simulink model "ATABEY_sistem_modeli"  (R2025b)
settings: Solver=VariableStepAuto  StartTime=0.0  StopTime=simTime  RelTol=1e-3
undefined symbols (not defined in the file or in its folder): uServoMax, x0
libraries: aerolibfltsims x1, aerolibanimutils x1
settings Model: Creator=erayacikgz  LastModifiedBy=erayacikgz

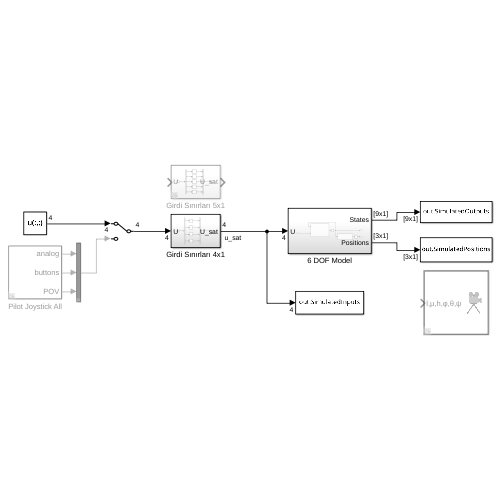
[thumbnail: Simulink's stored preview of the top-level diagram]
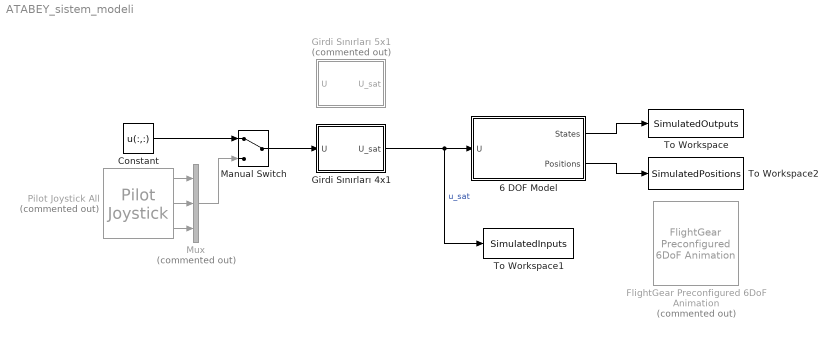
== system ATABEY_sistem_modeli ==
  6 DOF Model : Subsystem
  Constant : Constant  Value=u(:,:)
  FlightGear Preconfigured 6DoF Animation : aerolibfltsims/FlightGear Preconfigured 6DoF Animation  Commented=on  xFlightGearVersion=v2019.1  DestinationIpAddress=127.0.0.1  DestinationPort=5502  SampleTime=1/30  packetVersion=24
  Girdi Sınırları 4x1 : Subsystem
  Girdi Sınırları 5x1 : Subsystem  Commented=on
  Manual Switch : ManualSwitch
  Mux : Mux  Commented=on  Inputs=3
  Pilot Joystick All : aerolibanimutils/Pilot Joystick  Commented=on  JoystickID=Joystick1  OutputConfiguration=AllOutputs  SampleTime=1/30
      settings: LibrarySourceBlock=aerolibanimutils/Pilot Joystick All
  To Workspace : ToWorkspace  VariableName=SimulatedOutputs  SaveFormat=Timeseries  SampleTime=-1
  To Workspace1 : ToWorkspace  VariableName=SimulatedInputs  SaveFormat=Timeseries  SampleTime=-1
  To Workspace2 : ToWorkspace  VariableName=SimulatedPositions  SaveFormat=Timeseries  SampleTime=-1
  wires:
  6 DOF Model/1(States) -> To Workspace/1
  Constant/1 -> Manual Switch/1
  Pilot Joystick All/1 -> Mux/1
  Pilot Joystick All/2 -> Mux/2
  Pilot Joystick All/3 -> Mux/3
  Mux/1 -> Manual Switch/2
  6 DOF Model/2(Positions) -> To Workspace2/1
  Manual Switch/1 -> Girdi Sınırları 4x1/1(U)
  Girdi Sınırları 4x1/1(U_sat) -> To Workspace1/1, 6 DOF Model/1(U)  "u_sat"

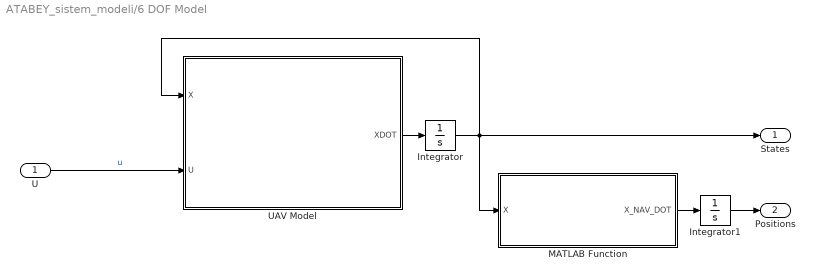
== system ATABEY_sistem_modeli/6 DOF Model ==
  U : Inport
  Integrator : Integrator  InitialCondition=x0(:,:)
  Integrator1 : Integrator  InitialCondition=[0;0;0;]
  MATLAB Function : MATLAB Function  TreatAsAtomicUnit=on
  UAV Model : MATLAB Function  TreatAsAtomicUnit=on
  States : Outport
  Positions : Outport  Port=2
  wires:
  U/1 -> UAV Model/2(U)  "u"
  UAV Model/1(XDOT) -> Integrator/1
  Integrator/1 -> UAV Model/1(X), States/1, MATLAB Function/1(X)
  MATLAB Function/1(X_NAV_DOT) -> Integrator1/1
  Integrator1/1 -> Positions/1

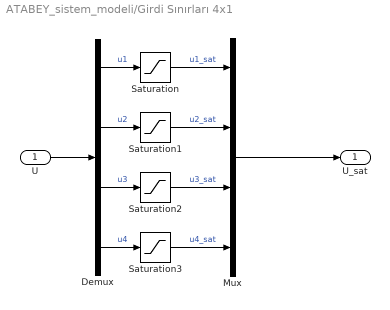
== system ATABEY_sistem_modeli/Girdi Sınırları 4x1 ==
  U : Inport
  Demux : Demux
  Mux : Mux
  Saturation : Saturate  UpperLimit=uServoMax  LowerLimit=-1*uServoMax
  Saturation1 : Saturate  UpperLimit=uServoMax  LowerLimit=-1*uServoMax
  Saturation2 : Saturate  UpperLimit=uServoMax  LowerLimit=-1*uServoMax
  Saturation3 : Saturate  UpperLimit=1  LowerLimit=0
  U_sat : Outport
  wires:
  Mux/1 -> U_sat/1
  Demux/2 -> Saturation1/1  "u2"
  Saturation/1 -> Mux/1  "u1_sat"
  Saturation2/1 -> Mux/3  "u3_sat"
  U/1 -> Demux/1
  Demux/1 -> Saturation/1  "u1"
  Demux/3 -> Saturation2/1  "u3"
  Saturation1/1 -> Mux/2  "u2_sat"
  Demux/4 -> Saturation3/1  "u4"
  Saturation3/1 -> Mux/4  "u4_sat"

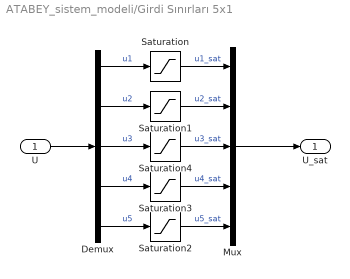
== system ATABEY_sistem_modeli/Girdi Sınırları 5x1 ==
  U : Inport
  Demux : Demux  Outputs=5
  Mux : Mux  Inputs=5
  Saturation : Saturate  UpperLimit=uServoMax  LowerLimit=-1*uServoMax
  Saturation1 : Saturate  UpperLimit=uServoMax  LowerLimit=-1*uServoMax
  Saturation2 : Saturate  UpperLimit=1  LowerLimit=0
  Saturation3 : Saturate  UpperLimit=1  LowerLimit=0
  Saturation4 : Saturate  UpperLimit=uServoMax  LowerLimit=-1*uServoMax
  U_sat : Outport
  wires:
  Mux/1 -> U_sat/1
  Demux/2 -> Saturation1/1  "u2"
  Saturation/1 -> Mux/1  "u1_sat"
  U/1 -> Demux/1
  Demux/1 -> Saturation/1  "u1"
  Saturation1/1 -> Mux/2  "u2_sat"
  Demux/4 -> Saturation3/1  "u4"
  Saturation3/1 -> Mux/4  "u4_sat"
  Demux/5 -> Saturation2/1  "u5"
  Saturation2/1 -> Mux/5  "u5_sat"
  Demux/3 -> Saturation4/1  "u3"
  Saturation4/1 -> Mux/3  "u3_sat"

== matlab function ATABEY_sistem_modeli/6 DOF Model/MATLAB Function ==
  data: X input; X_NAV_DOT output
function X_NAV_DOT  = NavigationEquations(X)

P_N_dot = X(1)*cos(X(8))*cos(X(9))...
    + X(2)*(-cos(X(7))*sin(X(9)) + sin(X(7))*sin(X(8))*cos(X(9)))...
    + X(3)*(sin(X(7))*sin(X(9)) + cos(X(7))*sin(X(8))*cos(X(9)));

P_E_dot = X(1)*cos(X(8))*sin(X(9))...
    + X(2)*(cos(X(7))*cos(X(9)) + sin(X(7))*sin(X(8))*sin(X(9)))...
    + X(3)*(-sin(X(7))*cos(X(9)) + cos(X(7))*sin(X(8))*sin(X(9)));

h_dot = X(1)*sin(X(8)) - X(2)*sin(X(7))*cos(X(8)) - X(3)*cos(X(7))*cos(X(8));

X_NAV_DOT = [P_N_dot;
             P_E_dot;
             h_dot];

end

== matlab function ATABEY_sistem_modeli/6 DOF Model/UAV Model ==
  data: X input double size=[9 1]; XDOT output double size=[9 1]; U input double
function XDOT = ATABEY_model(X, U)

    XDOT = ATABEY_dynamics(X, U);

end
